simulink model "Plano_Inicial_planta"  (R2018b)
settings: Solver=VariableStepAuto  StartTime=0.0  StopTime=10.0  RelTol=1e-3
values from neighbouring files (symbols this model uses):
  m = 0.0630    (= 0.063)    [ControleSimplificado.m]    (also in Plano_Piloto_trabalho.m)
settings Model: Creator=Adm  LastModifiedBy=Adm

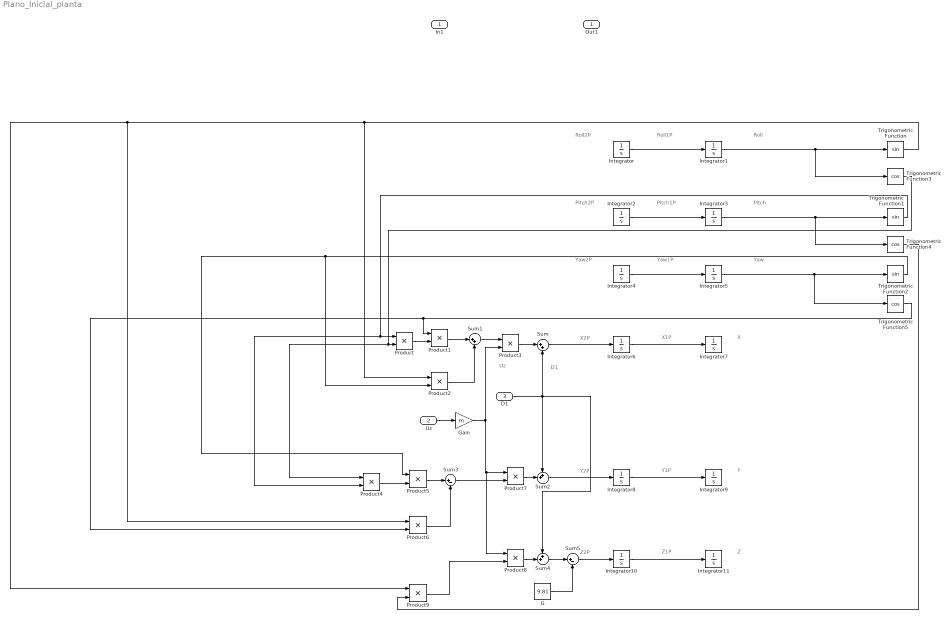
== system Plano_Inicial_planta ==
  note: D1
  note: Uz
  note: X2P
  note: X
  note: X1P
  note: Roll1P
  note: Roll
  note: Roll2P
  note: Pitch2P
  note: Pitch
  note: Pitch1P
  note: Yaw1P
  note: Yaw
  note: Yaw2P
  note: Y2P
  note: Y
  note: Y1P
  note: Z
  note: Z1P
  note: Z2P
  In1 : Inport
  Uz : Inport  Port=2
  D1 : Inport  Port=3
  G : Constant  Value=9.81
  Gain : Gain  Gain=m
  Integrator{,1..11} (12 alike) : Integrator
  Product{,1..9} (10 alike) : Product
  Sum : Sum  Inputs=|++
  Sum1 : Sum  Inputs=|++
  Sum2 : Sum  Inputs=++|
  Sum3 : Sum  Inputs=|+-
  Sum4 : Sum  Inputs=++|
  Sum5 : Sum  Inputs=|+-
  Trigonometric Function : Trigonometry
  Trigonometric Function1 : Trigonometry
  Trigonometric Function2 : Trigonometry
  Trigonometric Function3 : Trigonometry  Operator=cos
  Trigonometric Function4 : Trigonometry  Operator=cos
  Trigonometric Function5 : Trigonometry  Operator=cos
  Out1 : Outport
  wires:
  Integrator/1 -> Integrator1/1
  Integrator2/1 -> Integrator3/1
  Integrator4/1 -> Integrator5/1
  Integrator1/1 -> Trigonometric Function3/1, Trigonometric Function/1
  Integrator3/1 -> Trigonometric Function4/1, Trigonometric Function1/1
  Integrator5/1 -> Trigonometric Function5/1, Trigonometric Function2/1
  Integrator6/1 -> Integrator7/1
  Sum/1 -> Integrator6/1
  Trigonometric Function3/1 -> Product4/1, Product/2
  Trigonometric Function1/1 -> Product4/2, Product/1
  Product/1 -> Product1/2
  Trigonometric Function5/1 -> Product1/1, Product6/2
  Trigonometric Function2/1 -> Product5/1, Product2/2
  Product1/1 -> Sum1/1
  Product2/1 -> Sum1/2
  Sum1/1 -> Product3/1
  Product3/1 -> Sum/1
  D1/1 -> Sum4/1, Sum2/1, Sum/2
  Integrator8/1 -> Integrator9/1
  Sum2/1 -> Integrator8/1
  Product4/1 -> Product5/2
  Product5/1 -> Sum3/1
  Product6/1 -> Sum3/2
  Trigonometric Function/1 -> Product6/1, Product9/1, Product2/1
  Sum3/1 -> Product7/2
  Uz/1 -> Gain/1
  Gain/1 -> Product8/1, Product7/1, Product3/2
  Product7/1 -> Sum2/2
  Integrator10/1 -> Integrator11/1
  Product8/1 -> Sum4/2
  Product9/1 -> Product8/2
  Trigonometric Function4/1 -> Product9/2
  Sum5/1 -> Integrator10/1
  Sum4/1 -> Sum5/1
  G/1 -> Sum5/2
